simulink model "p2_1"  (R2021a)
settings: Solver=FixedStepAuto  StartTime=0.0  StopTime=inf  RelTol=1e-3  EnableMultiTasking=on
libraries: pil_lib x1
settings Model: SILPILModeSetting=veronly  CodeVerificationMode=processor-in-the-loop (pil)  EnablePacing=on  PacingRate=0.350000  ExtModeTrigDuration=2  Creator=Abbas  LastModifiedBy=Abbas
settings OptimizationCC: EnhancedBackFolding=on  PassReuseOutputArgsAs=Individual arguments  ZeroExternalMemoryAtStartup=off  ZeroInternalMemoryAtStartup=off  MaxStackSize=64  OptimizeBlockOrder=speed  DifferentSizesBufferReuse=on  OptimizationCustomize=off  EfficientTunableParamExpr=on
settings DebuggingCC: ParameterTunabilityLossMsg=error
settings HardwareCC: ProdBitPerInt=16  ProdBitPerPointer=16  ProdBitPerSizeT=16  ProdBitPerPtrDiffT=16  ProdLargestAtomicFloat=None  ProdWordSize=8  ProdHWDeviceType=Atmel->AVR
settings SFSimCC: MATLABDynamicMemAlloc=off
settings RTWCC: SystemTargetFile=ert.tlc  HardwareBoard=Arduino Mega 2560  TemplateMakefile=ert_default_tmf  Toolchain=Arduino AVR  BuildConfiguration=Faster Runs  CreateSILPILBlock=PIL
settings CodeAppCC: ForceParamTrailComments=on  IgnoreCustomStorageClasses=off  OperatorAnnotations=on  SimulinkDataObjDesc=on  SFDataObjDesc=on  InsertBlockDesc=on
settings ERTTargetCC: SupportContinuousTime=on  SupportVariableSizeSignals=on  ExtModeStaticAllocSize=2048

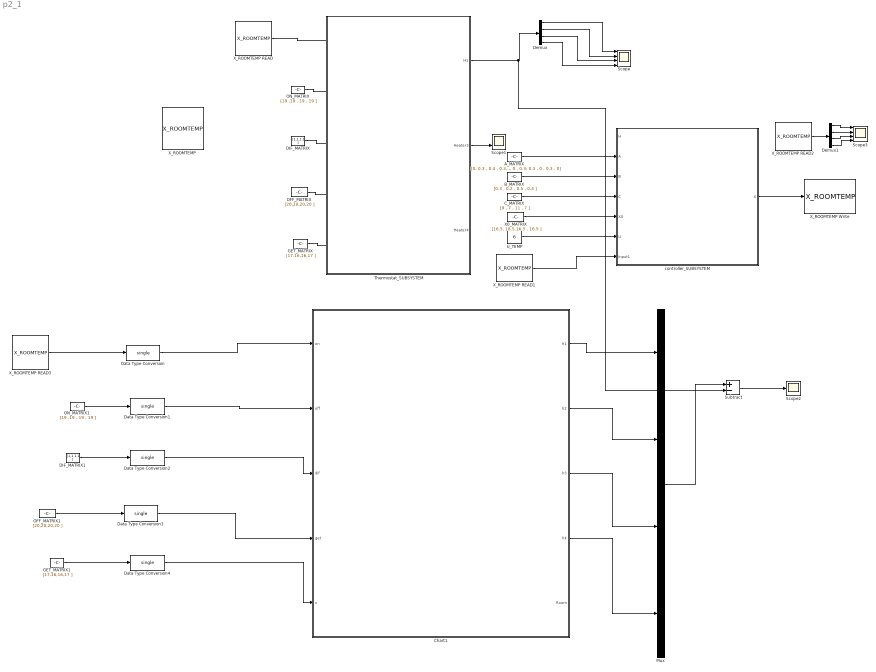
== system p2_1 ==
  A_MATRIX : Constant  Value=[0, 0.3 , 0.4 , 0.3 ; 0.3 , 0 , 0.5 , 0 ; 0.4 , 0.5 , 0 , 0.3; 0.3 , 0 , 0.3 , 0]
  B_MATRIX : Constant  Value=[0.3 , 0.2 , 0.5 , 0.4 ]
  C_MATRIX : Constant  Value=[9 , 7 , 11 , 7 ]
  Chart1 : Subsystem  DialogController=pil_create_dialog  LoadFcn=|
      | try
      |    if ~strcmp(rtw.pil.getPILVersion, '9.10 (R2021a)_15')
      |       set_param(gcb, 'DialogController', '');
      |       set_param(gcb, 'DialogControllerArgs', '');
      |    end
      | catch e
      |       set_param(gcb, 'DialogController', '');
      |       set_param(gcb, 'DialogControllerArgs', '');
      | end
      mask help: PIL:pil:XILBlockMaskDesc
      mask Display: disp('PIL');
  DIF_MATRIX : Constant  Value=[1,1,1,1 ]
  DIF_MATRIX1 : Constant  Value=[1,1,1,1 ]
  Data Type Conversion{,1..4} (5 alike) : DataTypeConversion  OutDataTypeStr=single
  Demux : Demux
  Demux1 : Demux
  GET_MATRIX : Constant  Value=[17,16,16,17 ]
  GET_MATRIX1 : Constant  Value=[17,16,16,17 ]
  Mux : Mux
  OFF_MATRIX : Constant  Value=[20,20,20,20 ]
  OFF_MATRIX1 : Constant  Value=[20,20,20,20 ]
  ON_MATRIX : Constant  Value=[19 ,19 , 19 , 19 ]
  ON_MATRIX1 : Constant  Value=[19 ,19 , 19 , 19 ]
  Scope : Scope  NumInputPorts=4
  Scope1 : Scope  NumInputPorts=2
  Scope2 : Scope
  Scope3 : Scope  NumInputPorts=4
  Subtract : Sum  Inputs=+-
  Thermostat_SUBSYSTEM : Subsystem
  U_TEMP : Constant  Value=6
  X0_MATRIX : Constant  Value=[16.5, 16.5,16.5 , 16.5 ]
  X_ROOMTEMP : DataStoreMemory  DataStoreName=X_ROOMTEMP  ReadBeforeWriteMsg=warning  WriteAfterWriteMsg=warning  WriteAfterReadMsg=warning  InitialValue=[16.5,16.5,16.5,16.5]  ShowAdditionalParam=off
  X_ROOMTEMP READ{,1..3} (4 alike) : DataStoreRead  DataStoreName=X_ROOMTEMP  IndexOptions=Index vector (dialog)  Indices=1  OutputSizes=1
  X_ROOMTEMP Write : DataStoreWrite  DataStoreName=X_ROOMTEMP  IndexOptions=Index vector (dialog)  Indices=1  OutputSizes=1
  controller_SUBSYSTEM : Subsystem
  wires:
  controller_SUBSYSTEM/1(X) -> X_ROOMTEMP Write/1
  X_ROOMTEMP READ/1 -> ?
  A_MATRIX/1 -> controller_SUBSYSTEM/2(A)
  B_MATRIX/1 -> controller_SUBSYSTEM/3(B)
  C_MATRIX/1 -> controller_SUBSYSTEM/4(C)
  X0_MATRIX/1 -> controller_SUBSYSTEM/5(X0)
  DIF_MATRIX/1 -> ?
  GET_MATRIX/1 -> ?
  OFF_MATRIX/1 -> ?
  ON_MATRIX/1 -> ?
  U_TEMP/1 -> controller_SUBSYSTEM/6(U)
  X_ROOMTEMP READ1/1 -> controller_SUBSYSTEM/7(Input1)
  Demux/1 -> Scope/1
  Demux/2 -> Scope/2
  Demux/3 -> Scope/3
  Demux/4 -> Scope/4
  Demux1/1 -> Scope3/1
  Demux1/2 -> Scope3/2
  Demux1/3 -> Scope3/3
  Demux1/4 -> Scope3/4
  X_ROOMTEMP READ2/1 -> Demux1/1
  Data Type Conversion1/1 -> Chart1/2(off)
  ON_MATRIX1/1 -> Data Type Conversion1/1
  GET_MATRIX1/1 -> Data Type Conversion4/1
  OFF_MATRIX1/1 -> Data Type Conversion3/1
  X_ROOMTEMP READ3/1 -> Data Type Conversion/1
  DIF_MATRIX1/1 -> Data Type Conversion2/1
  Data Type Conversion/1 -> Chart1/1(on)
  Mux/1 -> Subtract/1
  Subtract/1 -> Scope2/1
  Data Type Conversion2/1 -> Chart1/3(dif)
  Data Type Conversion3/1 -> Chart1/4(get)
  Data Type Conversion4/1 -> Chart1/5(x)
  Chart1/1(h1) -> Mux/1
  Chart1/2(h2) -> Mux/2
  Chart1/3(h3) -> Mux/3
  Thermostat_SUBSYSTEM/2(Heater3) -> Scope1/2
  Thermostat_SUBSYSTEM/1(H1) -> Subtract/2, Demux/1
  Chart1/4(h4) -> Mux/4

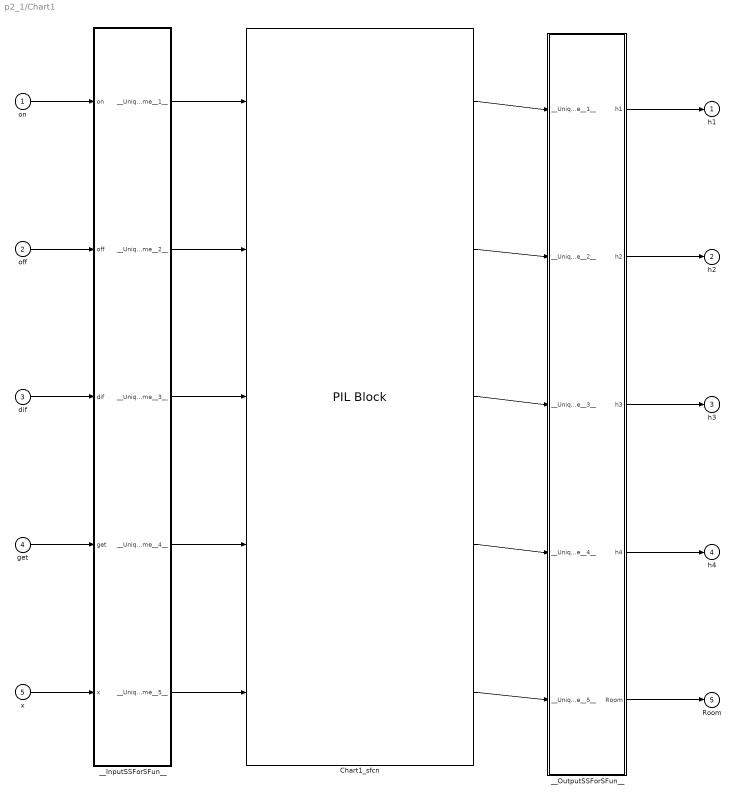
== system p2_1/Chart1 ==
  on : Inport
  off : Inport  Port=2
  dif : Inport  Port=3
  get : Inport  Port=4
  x : Inport  Port=5
  Chart1_sfcn : pil_lib/PIL Block  SimulationMode=PIL  IsTopModelPIL=off  CodeDir=C:\test2\Chart1_ert_rtw  AnchorDir=C:\test2  ConfigName=Arduino Board  XrelIsTopModelCode=on  XrelIsReusable=off  XrelDWorkNames={}  XrelDWorkTypes={}  XrelModelArgVals={}  XrelOrderedParamNames={}
      settings: SourceProductBaseCode=RT
  __InputSSForSFun__ : Subsystem
  __OutputSSForSFun__ : Subsystem
  h1 : Outport
  h2 : Outport  Port=2
  h3 : Outport  Port=3
  h4 : Outport  Port=4
  Room : Outport  Port=5
  wires:
  on/1 -> __InputSSForSFun__/1(on)
  off/1 -> __InputSSForSFun__/2(off)
  dif/1 -> __InputSSForSFun__/3(dif)
  get/1 -> __InputSSForSFun__/4(get)
  x/1 -> __InputSSForSFun__/5(x)
  __InputSSForSFun__/1(__UniqueOutportName__1__) -> Chart1_sfcn/1
  __InputSSForSFun__/2(__UniqueOutportName__2__) -> Chart1_sfcn/2
  __InputSSForSFun__/3(__UniqueOutportName__3__) -> Chart1_sfcn/3
  __InputSSForSFun__/4(__UniqueOutportName__4__) -> Chart1_sfcn/4
  __InputSSForSFun__/5(__UniqueOutportName__5__) -> Chart1_sfcn/5
  Chart1_sfcn/1 -> __OutputSSForSFun__/1(__UniqueInportName__1__)
  Chart1_sfcn/2 -> __OutputSSForSFun__/2(__UniqueInportName__2__)
  Chart1_sfcn/3 -> __OutputSSForSFun__/3(__UniqueInportName__3__)
  Chart1_sfcn/4 -> __OutputSSForSFun__/4(__UniqueInportName__4__)
  Chart1_sfcn/5 -> __OutputSSForSFun__/5(__UniqueInportName__5__)
  __OutputSSForSFun__/1(h1) -> h1/1
  __OutputSSForSFun__/2(h2) -> h2/1
  __OutputSSForSFun__/3(h3) -> h3/1
  __OutputSSForSFun__/4(h4) -> h4/1
  __OutputSSForSFun__/5(Room) -> Room/1

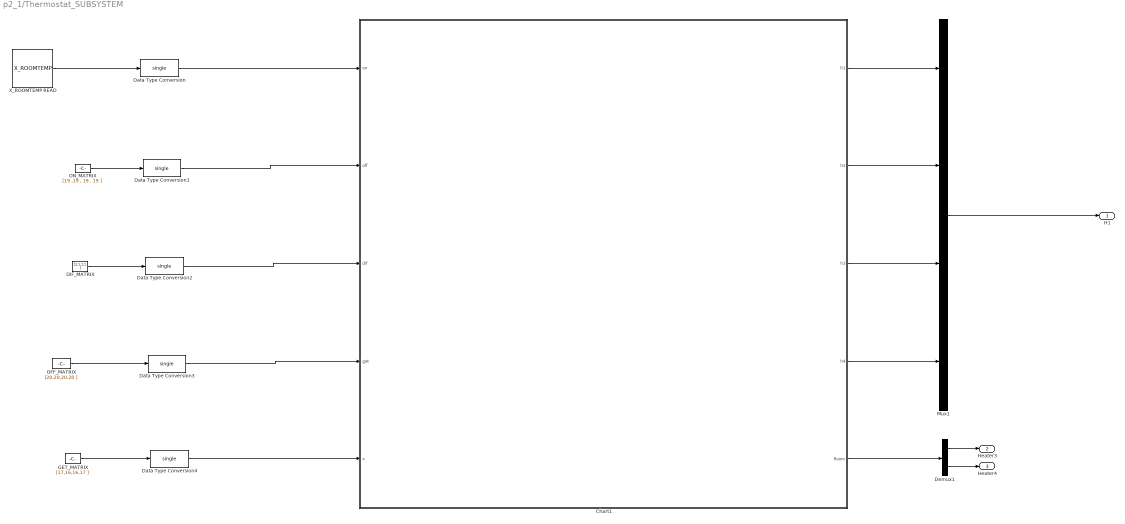
== system p2_1/Thermostat_SUBSYSTEM ==
  Chart1 : Stateflow chart  TreatAsAtomicUnit=on
      settings: MinAlgLoopOccurrences=on
  DIF_MATRIX : Constant  Value=[1,1,1,1 ]
  Data Type Conversion{,1..4} (5 alike) : DataTypeConversion  OutDataTypeStr=single
  Demux1 : Demux  Outputs=2
  GET_MATRIX : Constant  Value=[17,16,16,17 ]
  Mux1 : Mux
  OFF_MATRIX : Constant  Value=[20,20,20,20 ]
  ON_MATRIX : Constant  Value=[19 ,19 , 19 , 19 ]
  X_ROOMTEMP READ : DataStoreRead  DataStoreName=X_ROOMTEMP  IndexOptions=Index vector (dialog)  Indices=1  OutputSizes=1
  H1 : Outport
  Heater3 : Outport  Port=2
  Heater4 : Outport  Port=3
  wires:
  Mux1/1 -> H1/1
  Demux1/2 -> Heater4/1
  Demux1/1 -> Heater3/1
  Chart1/4(h4) -> Mux1/4
  Chart1/3(h3) -> Mux1/3
  Chart1/1(h1) -> Mux1/1
  Chart1/2(h2) -> Mux1/2
  Chart1/5(Room) -> Demux1/1
  Data Type Conversion4/1 -> Chart1/5(x)
  Data Type Conversion1/1 -> Chart1/2(off)
  ON_MATRIX/1 -> Data Type Conversion1/1
  GET_MATRIX/1 -> Data Type Conversion4/1
  Data Type Conversion2/1 -> Chart1/3(dif)
  Data Type Conversion3/1 -> Chart1/4(get)
  OFF_MATRIX/1 -> Data Type Conversion3/1
  X_ROOMTEMP READ/1 -> Data Type Conversion/1
  DIF_MATRIX/1 -> Data Type Conversion2/1
  Data Type Conversion/1 -> Chart1/1(on)

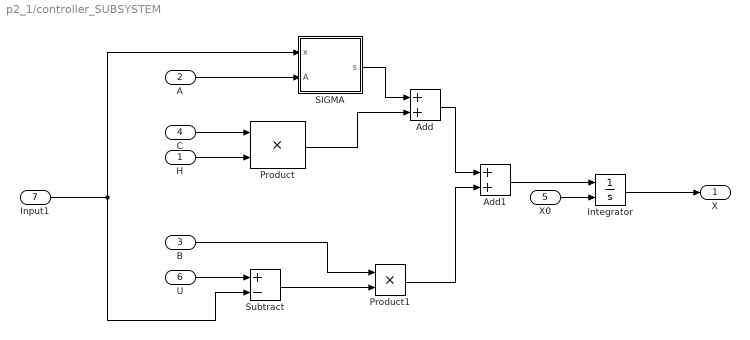
== system p2_1/controller_SUBSYSTEM ==
  H : Inport
  A : Inport  Port=2
  B : Inport  Port=3
  C : Inport  Port=4
  X0 : Inport  Port=5
  U : Inport  Port=6
  Input1 : Inport  Port=7
  Add : Sum
  Add1 : Sum
  Integrator : Integrator  InitialConditionSource=external
  Product : Product
  Product1 : Product
  SIGMA : Stateflow chart  TreatAsAtomicUnit=on
  Subtract : Sum  Inputs=+-
  X : Outport
  wires:
  C/1 -> Product/1
  H/1 -> Product/2
  U/1 -> Subtract/1
  B/1 -> Product1/1
  Subtract/1 -> Product1/2
  A/1 -> SIGMA/2(A)
  Product/1 -> Add/2
  SIGMA/1(s) -> Add/1
  Product1/1 -> Add1/2
  Add/1 -> Add1/1
  Add1/1 -> Integrator/1
  X0/1 -> Integrator/2
  Integrator/1 -> X/1
  Input1/1 -> SIGMA/1(x), Subtract/2

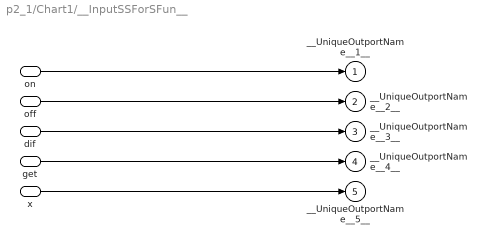
== system p2_1/Chart1/__InputSSForSFun__ ==
  on : Inport
  off : Inport  Port=2
  dif : Inport  Port=3
  get : Inport  Port=4
  x : Inport  Port=5
  __UniqueOutportName__1__ : Outport
  __UniqueOutportName__2__ : Outport  Port=2
  __UniqueOutportName__3__ : Outport  Port=3
  __UniqueOutportName__4__ : Outport  Port=4
  __UniqueOutportName__5__ : Outport  Port=5
  wires:
  on/1 -> __UniqueOutportName__1__/1
  off/1 -> __UniqueOutportName__2__/1
  dif/1 -> __UniqueOutportName__3__/1
  get/1 -> __UniqueOutportName__4__/1
  x/1 -> __UniqueOutportName__5__/1

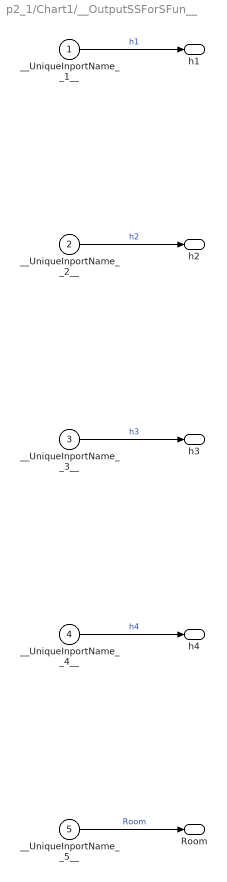
== system p2_1/Chart1/__OutputSSForSFun__ ==
  __UniqueInportName__1__ : Inport
  __UniqueInportName__2__ : Inport  Port=2
  __UniqueInportName__3__ : Inport  Port=3
  __UniqueInportName__4__ : Inport  Port=4
  __UniqueInportName__5__ : Inport  Port=5
  h1 : Outport
  h2 : Outport  Port=2
  h3 : Outport  Port=3
  h4 : Outport  Port=4
  Room : Outport  Port=5
  wires:
  __UniqueInportName__1__/1 -> h1/1  "h1"
  __UniqueInportName__2__/1 -> h2/1  "h2"
  __UniqueInportName__3__/1 -> h3/1  "h3"
  __UniqueInportName__4__/1 -> h4/1  "h4"
  __UniqueInportName__5__/1 -> Room/1  "Room"

== stateflow chart p2_1/Thermostat_SUBSYSTEM/Chart1 ==
  state st13
    entry:
    h2 = 0;
    h4 = 0;
    Room=[1,3];
    state s1 [parallel]
      settings: executionOrder=1
      state s1_on
        entry:
        h1 = 1
      state s1_off
        entry:
        h1 = 0
      (default) -> st13.s1.s1_on
      st13.s1.s1_on -> st13.s1.s1_off : [x(1)>=off(1)]
      st13.s1.s1_off -> st13.s1.s1_on : [x(1)<=on(1)]
    state s3 [parallel]
      settings: executionOrder=2
      state s3_on
        entry:
        h3 = 1
      state s3_off
        entry:
        h3 = 0
      (default) -> st13.s3.s3_on
      st13.s3.s3_on -> st13.s3.s3_off : [x(3)>=off(3)]
      st13.s3.s3_off -> st13.s3.s3_on : [x(3)<=on(3)]
  state st14
    entry:
    h2 = 0;
    h3 = 0;
    Room=[1,4];
    state s1 [parallel]
      settings: executionOrder=1
      state s1_on
        entry:
        h1 = 1
      state s1_off
        entry:
        h1 = 0
      (default) -> st14.s1.s1_on
      st14.s1.s1_on -> st14.s1.s1_off : [x(1)>=off(1)]
      st14.s1.s1_off -> st14.s1.s1_on : [x(1)<=on(1)]
    state s4 [parallel]
      settings: executionOrder=2
      state s4_on
        entry:
        h4 = 1
      state s4_off
        entry:
        h4 = 0
      (default) -> st14.s4.s4_on
      st14.s4.s4_on -> st14.s4.s4_off : [x(4)>=off(4)]
      st14.s4.s4_off -> st14.s4.s4_on : [x(4)<=on(4)]
  state st12
    entry:
    h3 = 0;
    h4 = 0;
    Room=[1,2];
    state s1 [parallel]
      settings: executionOrder=1
      state s1_on1
        entry:
        h1 = 1
      state s1_off
        entry:
        h1 = 0
      (default) -> s1_on1
      s1_on1 -> st12.s1.s1_off : [x(1)>=off(1) ]
      st12.s1.s1_off -> s1_on1 : [x(1)<=on(1) ]
    state s2 [parallel]
      settings: executionOrder=2
      state s2_on
        entry:
        h2 = 1
      state s1_off1
        entry:
        h2 = 0
      (default) -> st12.s2.s2_on
      st12.s2.s2_on -> s1_off1 : [x(2)>=off(2)]
      s1_off1 -> st12.s2.s2_on : [x(2)<=on(2)]
  state st24
    entry:
    h1 = 0;
    h3 = 0;
    Room=[1,3];
    state s2 [parallel]
      settings: executionOrder=1
      state s2_on
        entry:
        h2 = 1
      state s2_off
        entry:
        h2 = 0
      (default) -> st24.s2.s2_on
      st24.s2.s2_on -> s2_off : [x(2)>=off(2)]
      s2_off -> st24.s2.s2_on : [x(2)<=on(2)]
    state s4 [parallel]
      settings: executionOrder=2
      state s4_on
        entry:
        h4 = 1
      state s4_off
        entry:
        h4 = 0
      (default) -> st24.s4.s4_on
      st24.s4.s4_on -> st24.s4.s4_off : [x(4)>=off(4)]
      st24.s4.s4_off -> st24.s4.s4_on : [x(4)<=on(4)]
  state st34
    entry:
    h1 = 0;
    h2 = 0;
    Room=[3,4];
    state s3 [parallel]
      settings: executionOrder=1
      state s3_on
        entry:
        h3 = 1
      state s3_off
        entry:
        h3 = 0
      (default) -> st34.s3.s3_on
      st34.s3.s3_on -> st34.s3.s3_off : [x(3)>=off(3)]
      st34.s3.s3_off -> st34.s3.s3_on : [x(3)<=on(3)]
    state s4 [parallel]
      settings: executionOrder=2
      state s4_on
        entry:
        h4 = 1
      state s4_off
        entry:
        h4 = 0
      (default) -> st34.s4.s4_on
      st34.s4.s4_on -> st34.s4.s4_off : [x(4)>=off(4)]
      st34.s4.s4_off -> st34.s4.s4_on : [x(4)<=on(4)]
  state st23
    entry:
    h1 = 0;
    h4 = 0;
    Room=[2,3];
    state s2 [parallel]
      settings: executionOrder=1
      state s2_on
        entry:
        h2 = 1;
      state s1_off
        entry:
        h2 = 0;
      (default) -> st23.s2.s2_on
      st23.s2.s2_on -> st23.s2.s1_off : [x(2)>= off(2)]
      st23.s2.s1_off -> st23.s2.s2_on : [x(2)<=on(2)]
    state s3 [parallel]
      settings: executionOrder=2
      state s3_on
        entry:
        h3 = 1;
      state s3_off
        entry:
        h3 = 0;
      (default) -> st23.s3.s3_on
      st23.s3.s3_on -> st23.s3.s3_off : [x(3)>=off(3)]
      st23.s3.s3_off -> st23.s3.s3_on : [x(3)<=on(3) ]
  state start
    entry:
    h1=0
    h4=0
    h2=1;
    h3=1;
    Room=[2,3]
  st13 -> st14 [order 2] : [x(3)-x(4)>=dif(4) & x(4)<=get(4)]{h1=0;h3=0}
  st12 -> st13 [order 1] : [x(2)-x(3)>=dif(3) & x(3)<=get(3)]{h1=0;h2=0;}
  st13 -> st12 [order 1] : [x(3)-x(2)>=dif(2) & x(2)<=get(2)]{h1=0;h3=0;}
  st14 -> st13 [order 1] : [x(4)-x(3)>=dif(3) & x(3)<=get(3)]{h1=0;h4=0;}
  st13 -> st23 [order 3] : [(x(1)-x(2)>=dif(2) & x(2)<=get(2))]{h1=0;h3=0;}
  st13 -> st34 [order 4] : [x(1)-x(4)>=dif(4) & x(4)<=get(4)]{h1=0;h3=0;}
  st23 -> st13 [order 2] : [(x(2)-x(1)>=dif(1) & x(1)<=get(1))]{h2=0;h3=0}
  st34 -> st13 [order 1] : [x(4)-x(1)>=dif(1) & x(1)<=get(1)]{h3=0;h4=0;}
  st12 -> st14 [order 3] : [x(2)-x(4)>=dif(4) & x(4)<=get(4)]{h1=0;h2=0;}
  st14 -> st12 [order 2] : [x(4)-x(2)>=dif(2) & x(2)<=get(2)]{h1=0;h4=0;}
  st14 -> st24 [order 3] : [x(4)-x(2)>=dif(2) & x(2)<=get(2)]{h1=0;h4=0;}
  st24 -> st14 [order 2] : [x(2)-x(4)>=dif(4) & x(4)<=get(4)]{h2=0;h4=0;}
  st14 -> st34 [order 4] : [x(1)-x(3)>=dif(3) & x(3)<=get(3)]{h1=0;h4=0;}
  st34 -> st14 [order 2] : [x(3)-x(1)>=dif(1) & x(1)<=get(1)]{h3=0;h4=0;}
  st12 -> st23 [order 2] : [x(1)-x(3)>=dif(3) & x(3)<=get(3)]{h1=0;h2=0;}
  st23 -> st12 [order 1] : [x(3)-x(1)>=dif(1) & x(1)<=get(1)]{h2=0;h3=0;}
  st24 -> st12 [order 1] : [x(4)-x(1)>=dif(1) & x(1)<=get(1)]{h2=0;h4=0;}
  st12 -> st24 [order 4] : [x(1)-x(4)>=dif(4) & x(4)<=get(4)]{h1=0;h2=0;}
  (default) -> start
  start -> st23
  st23 -> st24 [order 3] : [x(3)-x(4)>=dif(4) & x(4)<=get(4)]{h2=0;h3=0;}
  st24 -> st34 [order 4] : [x(2)-x(3)>=dif(3) & x(3)<=get(3)]{h2=0;h4=0;}
  st24 -> st23 [order 3] : [x(4)-x(3)>=dif(3) & x(3)<=get(3)]{h2=0;h4=0;}
  st34 -> st24 [order 4] : [x(3)-x(2)>=dif(2) & x(2)<=get(2)]{h3=0;h4=0;}
  st23 -> st34 [order 4] : [x(2)-x(4)>=dif(4) & x(4)<=get(4)]{h3=0;h2=0;}
  st34 -> st23 [order 3] : [x(4)-x(2)>=dif(2) & x(2)<=get(2)]{h3=0;h4=0;}
  data: h1 output single; h2 output single; h3 output single; h4 output single; on input; off input; dif input; get input; x input single; Room output single

== stateflow chart p2_1/controller_SUBSYSTEM/SIGMA ==
  state s3
    du:
    s(1) = A(1,2)*(x(2)-x(1)) + A(1,3)*(x(3)-x(1)) + A(1,4)*(x(4)-x(1));
    s(2) = A(2,1)*(x(1)-x(2)) + A(2,3)*(x(3)-x(2)) + A(2,4)*(x(4)-x(2));
    s(3) = A(3,1)*(x(1)-x(3)) + A(3,2)*(x(2)-x(3)) + A(3,4)*(x(4)-x(3));
    s(4) = A(4,1)*(x(1)-x(4)) + A(4,2)*(x(2)-x(4)) + A(4,3)*(x(3)-x(4));
  (default) -> s3 : {s=[0,0,0,0];}
  data: x input; A input; s output
